simulink model "Project_Simulink_April15"  (R2019b)
settings: Solver=FixedStepAuto  StartTime=0.0  StopTime=6  FixedStep=0.005  RelTol=1e-3
StopFcn:
  | Project_Simulink_Plotz_April15
values from neighbouring files (symbols this model uses):
  cf = 750    [Project_Simulink_Params_April15.m]
  cr = 750    [Project_Simulink_Params_April15.m]
  Cr_ext = 750    [Project_Simulink_Params_April15.m]
  Delay = L/V    [Project_Simulink_Params_April15.m]
  FG = 1.35    [Project_Simulink_Params_April15.m]
  Iyy = 82    [Project_Simulink_Params_April15.m]
  kf = 2190    [Project_Simulink_Params_April15.m]
  kr = 3365    [Project_Simulink_Params_April15.m]
  L = Lf + Lr    (= 1.422)    [Project_Simulink_Params_April15.m]
  Lf = 0.64    [Project_Simulink_Params_April15.m]
  Lr = 0.782    [Project_Simulink_Params_April15.m]
  Mb = 193    [Project_Simulink_Params_April15.m]
  OG = 0.60    (= 0.6)    [Project_Simulink_Params_April15.m]
  RampEnd = cosd(Angle)* RampLength/V + RampStart    [Project_Simulink_Params_April15.m]
  RampStart = 2    [Project_Simulink_Params_April15.m]
  RDG1 = 0.4    [Project_Simulink_Params_April15.m]
  RDG2 = 1    [Project_Simulink_Params_April15.m]
  RSG1 = 0.75    [Project_Simulink_Params_April15.m]
  RSG2 = 0.75    [Project_Simulink_Params_April15.m]
  Ts = 0.005    [Project_Simulink_Params_April15.m]
  V = Vs(i)    [Project_Simulink_Params_April15.m]
libraries: commfilt2 x5, simulink x2, dspsigops x1
settings Model: Creator=Jordan  LastModifiedBy=Jordan
settings DataIOCC: SaveFormat=Array  ReturnWorkspaceOutputs=off
settings DebuggingCC: ArithmeticOperatorsInVariantConditions=warning
settings SFSimCC: SimUseLocalCustomCode=off  CustomCodeUndefinedFunction=UseInterfaceOnly
settings RTWCC: RTWUseLocalCustomCode=off

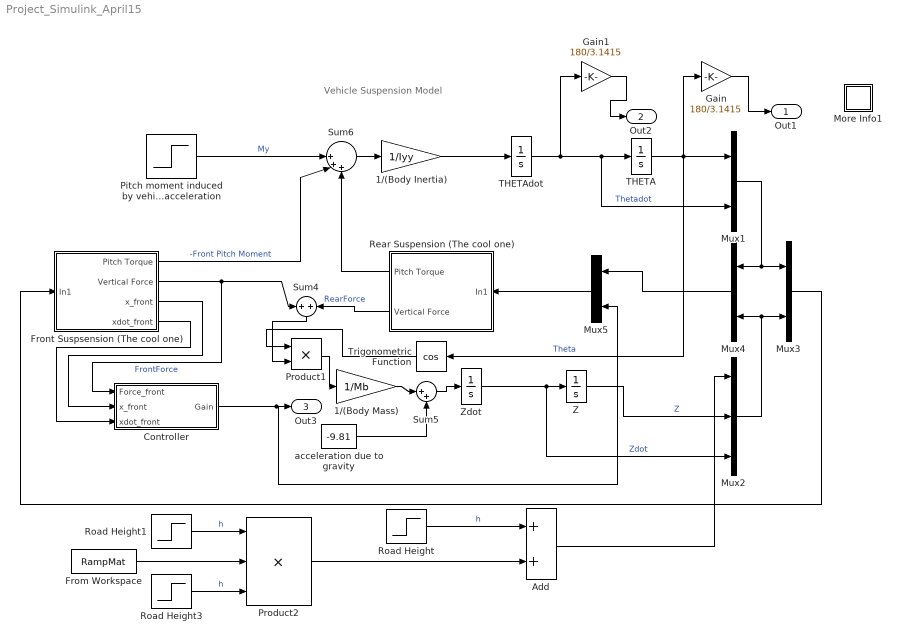
== system Project_Simulink_April15 ==
  note: Vehicle Suspension Model
  1/(Body Inertia) : Gain  Gain=1/Iyy  SaturateOnIntegerOverflow=on  OutDataTypeStr=Inherit: Same as input  ParamDataTypeStr=Inherit: Same as input
  1/(Body Mass) : Gain  Gain=1/Mb  SaturateOnIntegerOverflow=on  OutDataTypeStr=Inherit: Same as input  ParamDataTypeStr=Inherit: Same as input
  Add : Sum
  Controller : Subsystem
  From Workspace : FromWorkspace  VariableName=RampMat  OutputAfterFinalValue=Holding final value
  Front Suspsension (The cool one) : Subsystem
  Gain : Gain  Gain=180/3.1415
  Gain1 : Gain  Gain=180/3.1415
  More Info1 : Subsystem
      settings: OpenFcn=showdemo(bdroot(gcb))
      mask Display: disp('?')
  Mux{1,3..5} (4 alike) : Mux  Inputs=2
      settings: DisplayOption=signals
  Mux2 : Mux  Inputs=3
      settings: DisplayOption=signals
  Pitch moment induced by vehicle acceleration : Step  Time=3  After=0  SampleTime=0
  Product1 : Product
  Product2 : Product  Inputs=3
  Rear Suspension (The cool one) : Subsystem
  Road Height : Step  Time=0  After=0  SampleTime=0
  Road Height1 : Step  Time=RampStart  SampleTime=0
  Road Height3 : Step  Time=RampEnd  Before=1  After=0  SampleTime=0
  Sum4 : Sum  SaturateOnIntegerOverflow=on  InputSameDT=on  OutDataTypeStr=Inherit: Same as first input
  Sum5 : Sum  Inputs=|++  SaturateOnIntegerOverflow=on  InputSameDT=on  OutDataTypeStr=Inherit: Same as first input
  Sum6 : Sum  Inputs=||+++  SaturateOnIntegerOverflow=on  InputSameDT=on  OutDataTypeStr=Inherit: Same as first input
  THETA : Integrator  InitialCondition=5*3.1415/180
  THETAdot : Integrator  InitialCondition=8.04e-28
  Trigonometric Function : Trigonometry  Operator=cos
  Z : Integrator  InitialCondition=-0.12
  Zdot : Integrator
  acceleration due to gravity : Constant  Value=-9.81
  Out1 : Outport
  Out2 : Outport  Port=2
  Out3 : Outport  Port=3
  wires:
  acceleration due to gravity/1 -> Sum5/2
  1/(Body Mass)/1 -> Sum5/1
  1/(Body Inertia)/1 -> THETAdot/1
  Zdot/1 -> Mux2/3, Z/1  "Zdot"
  Z/1 -> Mux2/2  "Z"
  Front Suspsension (The cool one)/1(Pitch Torque) -> Sum6/2  "-Front Pitch Moment"
  Mux3/1 -> Front Suspsension (The cool one)/1(In1)
  Rear Suspension (The cool one)/2(Vertical Force) -> Sum4/2  "RearForce"
  Mux2/1 -> Mux4/2, Mux3/2
  Rear Suspension (The cool one)/1(Pitch Torque) -> Sum6/3
  Pitch moment induced by vehicle acceleration/1 -> Sum6/1  "My"
  Sum6/1 -> 1/(Body Inertia)/1
  THETAdot/1 -> Gain1/1, THETA/1, Mux1/2  "Thetadot"
  THETA/1 -> Trigonometric Function/1, Gain/1, Mux1/1  "Theta"
  Front Suspsension (The cool one)/2(Vertical Force) -> Controller/1(Force_front), Sum4/1  "FrontForce"
  Sum5/1 -> Zdot/1
  Mux1/1 -> Mux3/1, Mux4/1
  Road Height/1 -> Add/1  "h"
  Add/1 -> Mux2/1
  Gain1/1 -> Out2/1
  Front Suspsension (The cool one)/3(x_front) -> Controller/2(x_front)
  Front Suspsension (The cool one)/4(xdot_front) -> Controller/3(xdot_front)
  Mux4/1 -> Mux5/1
  Controller/1("Gain ") -> Mux5/2, Out3/1
  Mux5/1 -> Rear Suspension (The cool one)/1(In1)
  Gain/1 -> Out1/1
  Trigonometric Function/1 -> Product1/1
  Sum4/1 -> Product1/2
  Product1/1 -> 1/(Body Mass)/1
  Road Height3/1 -> Product2/3  "h"
  From Workspace/1 -> Product2/2
  Road Height1/1 -> Product2/1  "h"
  Product2/1 -> Add/2

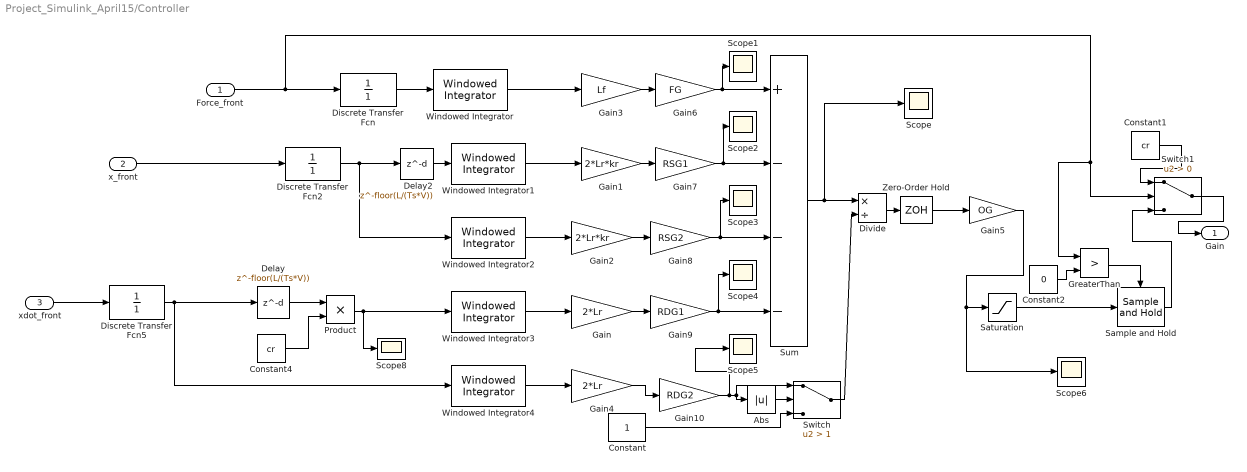
== system Project_Simulink_April15/Controller ==
  Force_front : Inport
  x_front : Inport  Port=2
  xdot_front : Inport  Port=3
  Abs : Abs
  Constant : Constant
  Constant1 : Constant  Value=cr
  Constant2 : Constant  Value=0
  Constant4 : Constant  Value=cr
  Delay : Delay  DelayLength=floor(L/(Ts*V))  SampleTime=Ts
  Delay2 : Delay  DelayLength=floor(L/(Ts*V))  SampleTime=Ts
  Discrete Transfer Fcn : DiscreteTransferFcn  Denominator=[1]  SampleTime=Ts
  Discrete Transfer Fcn2 : DiscreteTransferFcn  Denominator=[1]  SampleTime=Ts
  Discrete Transfer Fcn5 : DiscreteTransferFcn  Denominator=[1]  SampleTime=Ts
  Divide : Product  Inputs=*/
  Gain : Gain  Gain=2*Lr
  Gain1 : Gain  Gain=2*Lr*kr
  Gain10 : Gain  Gain=RDG2
  Gain2 : Gain  Gain=2*Lr*kr
  Gain3 : Gain  Gain=Lf
  Gain4 : Gain  Gain=2*Lr
  Gain5 : Gain  Gain=OG
  Gain6 : Gain  Gain=FG
  Gain7 : Gain  Gain=RSG1
  Gain8 : Gain  Gain=RSG2
  Gain9 : Gain  Gain=RDG1
  GreaterThan : RelationalOperator  Operator=>  OutDataTypeStr=boolean  RndMeth=Simplest
  Product : Product
  Sample and Hold : dspsigops/Sample and Hold  trig=Falling edge  initCond=0  latchinput=off
  Saturation : Saturate  UpperLimit=750  LowerLimit=750
  Scope{,1..6,8} (8 alike) : Scope
  Sum : Sum  Inputs=+---
  Switch : Switch  Criteria=u2 > Threshold  Threshold=1
  Switch1 : Switch  Criteria=u2 > Threshold
  Windowed Integrator{,1..4} (5 alike) : commfilt2/Windowed Integrator  integperiod=floor(L/(Ts*V))  InputProcessing=Columns as channels (frame based)  roundingMode=Floor  overflowMode=off  coeffDataTypeStr=Inherit: Same word length as input  coeffMin=[]  coeffMax=[]  coeffLastDataTypeStr=Inherit: Same word length as input  accumDataTypeStr=Inherit: Same as product output  accumLastDataTypeStr=Inherit: Same as product output  outputDataTypeStr=Inherit: Same as accumulator  outputMin=[]  outputMax=[]  outputLastDataTypeStr=Inherit: Same as accumulator
      settings: SourceProductName=Communications Toolbox  SourceProductBaseCode=CM
  Zero-Order Hold : ZeroOrderHold  SampleTime=Ts
  "Gain " : Outport
  wires:
  Force_front/1 -> GreaterThan/1, Switch1/2, Discrete Transfer Fcn/1
  Windowed Integrator/1 -> Gain3/1
  Delay/1 -> Product/1
  Sum/1 -> Scope/1, Divide/1
  Divide/1 -> Zero-Order Hold/1
  Windowed Integrator1/1 -> Gain1/1
  Windowed Integrator2/1 -> Gain2/1
  Windowed Integrator3/1 -> Gain/1
  Windowed Integrator4/1 -> Gain4/1
  Discrete Transfer Fcn/1 -> Windowed Integrator/1
  x_front/1 -> Discrete Transfer Fcn2/1
  Discrete Transfer Fcn2/1 -> Windowed Integrator2/1, Delay2/1
  Product/1 -> Windowed Integrator3/1, Scope8/1
  xdot_front/1 -> Discrete Transfer Fcn5/1
  Zero-Order Hold/1 -> Gain5/1
  Gain4/1 -> Gain10/1
  Switch/1 -> Divide/2
  Abs/1 -> Switch/2
  Constant/1 -> Switch/3
  Delay2/1 -> Windowed Integrator1/1
  Discrete Transfer Fcn5/1 -> Windowed Integrator4/1, Delay/1
  Switch1/1 -> "Gain "/1
  Constant1/1 -> Switch1/1
  GreaterThan/1 -> Sample and Hold/Trigger
  Constant2/1 -> GreaterThan/2
  Sample and Hold/1 -> Switch1/3
  Constant4/1 -> Product/2
  Saturation/1 -> Sample and Hold/1
  Gain3/1 -> Gain6/1
  Gain6/1 -> Scope1/1, Sum/1
  Gain1/1 -> Gain7/1
  Gain7/1 -> Scope2/1, Sum/2
  Gain2/1 -> Gain8/1
  Gain8/1 -> Scope3/1, Sum/3
  Gain9/1 -> Scope4/1, Sum/4
  Gain/1 -> Gain9/1
  Gain10/1 -> Scope5/1, Abs/1, Switch/1
  Gain5/1 -> Scope6/1, Saturation/1

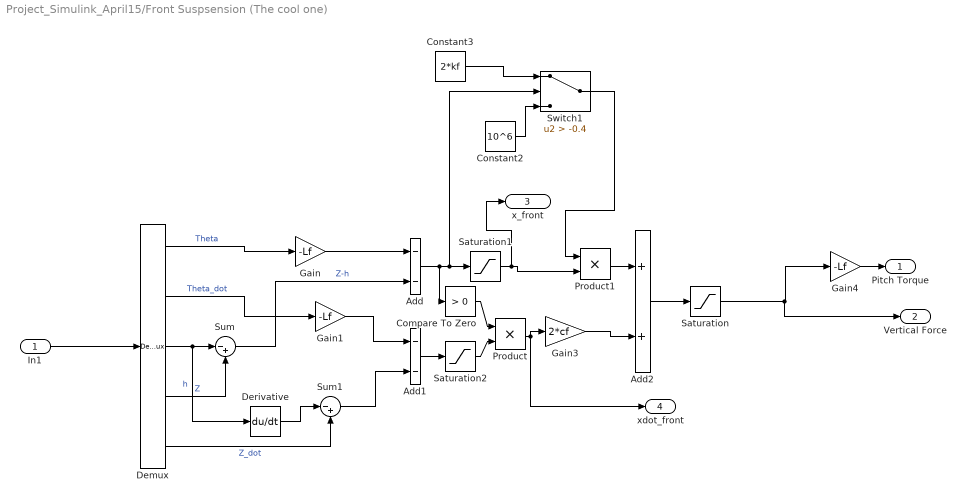
== system Project_Simulink_April15/Front Suspsension (The cool one) ==
  In1 : Inport
  Add : Sum  Inputs=--
  Add1 : Sum  Inputs=--
  Add2 : Sum
  Compare To Zero : simulink/Logic and Bit Operations/Compare To Zero  relop=>  OutDataTypeStr=boolean
  Constant2 : Constant  Value=10^6
  Constant3 : Constant  Value=2*kf
  Demux : Demux  Outputs=5
  Derivative : Derivative
  Gain : Gain  Gain=-Lf
  Gain1 : Gain  Gain=-Lf
  Gain3 : Gain  Gain=2*cf
  Gain4 : Gain  Gain=-Lf
  Product : Product
  Product1 : Product
  Saturation : Saturate  UpperLimit=inf  LowerLimit=0
  Saturation1 : Saturate  UpperLimit=inf  LowerLimit=0
  Saturation2 : Saturate  UpperLimit=inf  LowerLimit=-5
  Sum : Sum  Inputs=|-+
  Sum1 : Sum  Inputs=|-+
  Switch1 : Switch  Criteria=u2 > Threshold  Threshold=-0.4
  Pitch Torque : Outport  VectorParamsAs1DForOutWhenUnconnected=off
  Vertical Force : Outport  Port=2  VectorParamsAs1DForOutWhenUnconnected=off
  x_front : Outport  Port=3  VectorParamsAs1DForOutWhenUnconnected=off
  xdot_front : Outport  Port=4  VectorParamsAs1DForOutWhenUnconnected=off
  wires:
  In1/1 -> Demux/1
  Demux/1 -> Gain/1  "Theta"
  Demux/2 -> Gain1/1  "Theta_dot"
  Gain/1 -> Add/1
  Gain1/1 -> Add1/1
  Add/1 -> Switch1/2, Saturation1/1, Compare To Zero/1
  Gain4/1 -> Pitch Torque/1
  Add2/1 -> Saturation/1
  Demux/4 -> Sum/2  "Z"
  Demux/3 -> Derivative/1, Sum/1  "h"
  Sum/1 -> Add/2  "Z-h"
  Saturation/1 -> Vertical Force/1, Gain4/1
  Derivative/1 -> Sum1/1
  Demux/5 -> Sum1/2  "Z_dot"
  Sum1/1 -> Add1/2
  Product/1 -> xdot_front/1, Gain3/1
  Compare To Zero/1 -> Product/1
  Product1/1 -> Add2/1
  Gain3/1 -> Add2/2
  Add1/1 -> Saturation2/1
  Saturation2/1 -> Product/2
  Switch1/1 -> Product1/1
  Saturation1/1 -> x_front/1, Product1/2
  Constant2/1 -> Switch1/3
  Constant3/1 -> Switch1/1

== system Project_Simulink_April15/More Info1 ==

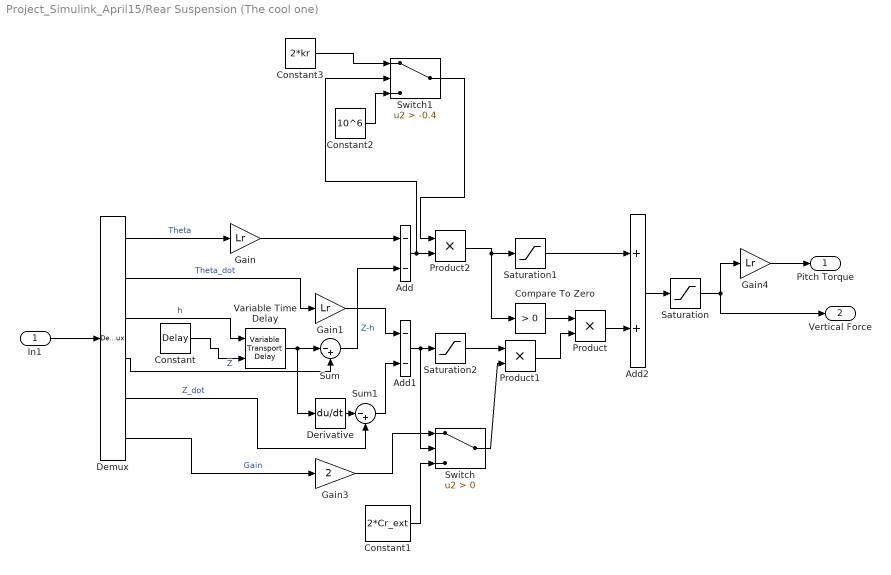
== system Project_Simulink_April15/Rear Suspension (The cool one) ==
  In1 : Inport
  Add : Sum  Inputs=--
  Add1 : Sum  Inputs=--
  Add2 : Sum
  Compare To Zero : simulink/Logic and Bit Operations/Compare To Zero  relop=>  OutDataTypeStr=boolean
  Constant : Constant  Value=Delay
  Constant1 : Constant  Value=2*Cr_ext
  Constant2 : Constant  Value=10^6
  Constant3 : Constant  Value=2*kr
  Demux : Demux  Outputs=6
  Derivative : Derivative
  Gain : Gain  Gain=Lr
  Gain1 : Gain  Gain=Lr
  Gain3 : Gain  Gain=2
  Gain4 : Gain  Gain=Lr
  Product : Product
  Product1 : Product
  Product2 : Product
  Saturation : Saturate  UpperLimit=inf  LowerLimit=0
  Saturation1 : Saturate  UpperLimit=inf  LowerLimit=0
  Saturation2 : Saturate  UpperLimit=inf  LowerLimit=-5
  Sum : Sum  Inputs=|-+
  Sum1 : Sum  Inputs=|-+
  Switch : Switch  Criteria=u2 > Threshold
  Switch1 : Switch  Criteria=u2 > Threshold  Threshold=-0.4
  Variable Time Delay : VariableTransportDelay  MaximumDelay=10
  Pitch Torque : Outport  VectorParamsAs1DForOutWhenUnconnected=off
  Vertical Force : Outport  Port=2  VectorParamsAs1DForOutWhenUnconnected=off
  wires:
  In1/1 -> Demux/1
  Demux/1 -> Gain/1  "Theta"
  Demux/2 -> Gain1/1  "Theta_dot"
  Gain/1 -> Add/1
  Gain1/1 -> Add1/1
  Product2/1 -> Saturation1/1, Compare To Zero/1
  Gain4/1 -> Pitch Torque/1
  Add2/1 -> Saturation/1
  Demux/4 -> Sum/2  "Z"
  Sum/1 -> Add/2  "Z-h"
  Variable Time Delay/1 -> Derivative/1, Sum/1
  Demux/3 -> Variable Time Delay/1  "h"
  Constant/1 -> Variable Time Delay/2
  Saturation/1 -> Vertical Force/1, Gain4/1
  Saturation1/1 -> Add2/1
  Demux/5 -> Sum1/2  "Z_dot"
  Derivative/1 -> Sum1/1
  Sum1/1 -> Add1/2
  Compare To Zero/1 -> Product/1
  Product/1 -> Add2/2
  Add1/1 -> Switch/2, Saturation2/1
  Demux/6 -> Gain3/1  "Gain"
  Product1/1 -> Product/2
  Saturation2/1 -> Product1/1
  Gain3/1 -> Switch/1
  Switch/1 -> Product1/2
  Constant1/1 -> Switch/3
  Constant3/1 -> Switch1/1
  Switch1/1 -> Product2/1
  Constant2/1 -> Switch1/3
  Add/1 -> Product2/2, Switch1/2
